simulink model "ex1"  (R2016a)
settings: Solver=VariableStepAuto  StartTime=0.0  StopTime=10.0  RelTol=1e-3
settings Model: Creator=Utilizator  LastModifiedBy=Utilizator

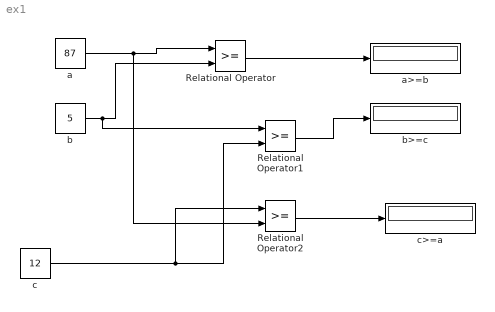
== system ex1 ==
  Relational Operator : RelationalOperator  OutDataTypeStr=boolean
  Relational Operator1 : RelationalOperator  OutDataTypeStr=boolean
  Relational Operator2 : RelationalOperator  OutDataTypeStr=boolean
  a : Constant  Value=87
  a>=b : Display
  b : Constant  Value=5
  b>=c : Display
  c : Constant  Value=12
  c>=a : Display
  wires:
  a/1 -> Relational Operator2/2, Relational Operator/1
  b/1 -> Relational Operator1/1, Relational Operator/2
  c/1 -> Relational Operator2/1, Relational Operator1/2
  Relational Operator/1 -> a>=b/1
  Relational Operator1/1 -> b>=c/1
  Relational Operator2/1 -> c>=a/1
